simulink model "Adaptive_Cruise_Control"  (R2022b)
settings: configuration reference "CommonModelConfiguration" (kept outside this file)
undefined symbols (not defined in the file): cc_param_23, LCFG_ACC_IntStsDelay, LCFG_ACC_Tmr1, LCFG_ACC_Tmr2, LCFG_ActivationDeactivation, LCFG_DSF_Timeout
settings Model: Creator=rkallum  LastModifiedBy=OTHOMSO1
settings ConfigSetRef: SourceName=CommonModelConfiguration  SourceLocation=Base Workspace

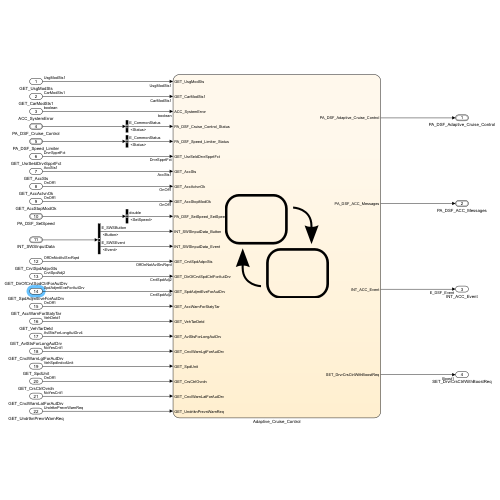
[thumbnail: Simulink's stored preview of the top-level diagram]
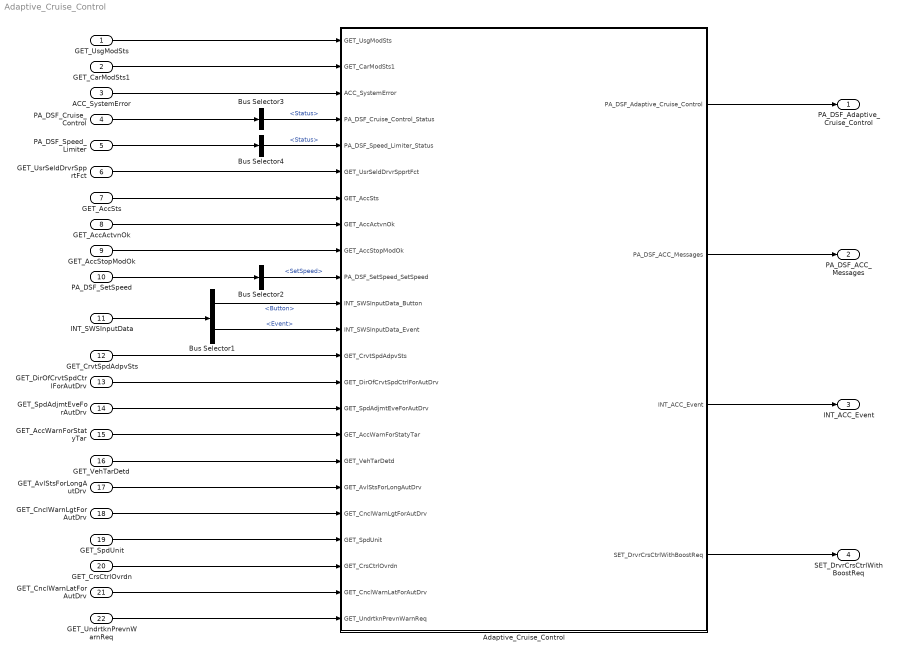
== system Adaptive_Cruise_Control ==
  GET_UsgModSts : Inport  OutDataTypeStr=Enum: UsgModSts1
  GET_CarModSts1 : Inport  Port=2  OutDataTypeStr=Enum: CarModSts1
  ACC_SystemError : Inport  Port=3  OutDataTypeStr=boolean
  PA_DSF_Cruise_Control : Inport  Port=4  OutDataTypeStr=Bus: PA_DSF
  PA_DSF_Speed_Limiter : Inport  Port=5  OutDataTypeStr=Bus: PA_DSF
  GET_UsrSeldDrvrSpprtFct : Inport  Port=6  OutDataTypeStr=Enum: DrvrSpprtFct
  GET_AccSts : Inport  Port=7  OutDataTypeStr=Enum: AccSts1
  GET_AccActvnOk : Inport  Port=8  OutDataTypeStr=Enum: OnOff1
  GET_AccStopModOk : Inport  Port=9  OutDataTypeStr=Enum: OnOff1
  PA_DSF_SetSpeed : Inport  Port=10  OutDataTypeStr=Bus: PA_StatusAndValueAndDoubleAndDouble
  INT_SWSInputData : Inport  Port=11  OutDataTypeStr=Bus: SWSInputData  LockScale=on
  GET_CrvtSpdAdpvSts : Inport  Port=12  OutDataTypeStr=Enum: OffOnNotAvlSrvRqrd
  GET_DirOfCrvtSpdCtrlForAutDrv : Inport  Port=13  OutDataTypeStr=Enum: CrvtSpdAdj2
  GET_SpdAdjmtEveForAutDrv : Inport  Port=14  OutDataTypeStr=Enum: SpdAdjmtEveForAutDrv
  GET_AccWarnForStatyTar : Inport  Port=15  OutDataTypeStr=Enum: OnOff1
  GET_VehTarDetd : Inport  Port=16  OutDataTypeStr=Enum: VehDetd1
  GET_AvlStsForLongAutDrv : Inport  Port=17  OutDataTypeStr=Enum: AvlStsForLongAutDrv4
  GET_CnclWarnLgtForAutDrv : Inport  Port=18  OutDataTypeStr=Enum: NoYesCrit1
  GET_SpdUnit : Inport  Port=19  OutDataTypeStr=Enum: VehSpdIndcdUnit
  GET_CrsCtrlOvrdn : Inport  Port=20  OutDataTypeStr=Enum: OnOff1
  GET_CnclWarnLatForAutDrv : Inport  Port=21  OutDataTypeStr=Enum: NoYesCrit1
  GET_UndrtknPrevnWarnReq : Inport  Port=22  OutDataTypeStr=Enum: UndrtknPrevnWarnReq
  Adaptive_Cruise_Control : Stateflow chart  TreatAsAtomicUnit=on
  Bus Selector1 : BusSelector  OutputSignals=Button,Event
  Bus Selector2 : BusSelector  OutputSignals=SetSpeed
  Bus Selector3 : BusSelector  OutputSignals=Status
  Bus Selector4 : BusSelector  OutputSignals=Status
  PA_DSF_Adaptive_Cruise_Control : Outport  OutDataTypeStr=Bus: PA_DSF_ACC  VectorParamsAs1DForOutWhenUnconnected=off
  PA_DSF_ACC_Messages : Outport  Port=2  OutDataTypeStr=Bus: PA_DSF_Message  VectorParamsAs1DForOutWhenUnconnected=off
  INT_ACC_Event : Outport  Port=3  OutDataTypeStr=Enum: E_DSF_Event  VectorParamsAs1DForOutWhenUnconnected=off
  SET_DrvrCrsCtrlWithBoostReq : Outport  Port=4  OutDataTypeStr=Enum: Boost1  VectorParamsAs1DForOutWhenUnconnected=off
  wires:
  ACC_SystemError/1 -> Adaptive_Cruise_Control/3(ACC_SystemError)
  PA_DSF_Cruise_Control/1 -> Bus Selector3/1
  PA_DSF_Speed_Limiter/1 -> Bus Selector4/1
  GET_UsrSeldDrvrSpprtFct/1 -> Adaptive_Cruise_Control/6(GET_UsrSeldDrvrSpprtFct)
  GET_AccSts/1 -> Adaptive_Cruise_Control/7(GET_AccSts)
  GET_AccActvnOk/1 -> Adaptive_Cruise_Control/8(GET_AccActvnOk)
  GET_AccStopModOk/1 -> Adaptive_Cruise_Control/9(GET_AccStopModOk)
  PA_DSF_SetSpeed/1 -> Bus Selector2/1
  GET_CrvtSpdAdpvSts/1 -> Adaptive_Cruise_Control/13(GET_CrvtSpdAdpvSts)
  GET_DirOfCrvtSpdCtrlForAutDrv/1 -> Adaptive_Cruise_Control/14(GET_DirOfCrvtSpdCtrlForAutDrv)
  GET_AccWarnForStatyTar/1 -> Adaptive_Cruise_Control/16(GET_AccWarnForStatyTar)
  GET_VehTarDetd/1 -> Adaptive_Cruise_Control/17(GET_VehTarDetd)
  GET_AvlStsForLongAutDrv/1 -> Adaptive_Cruise_Control/18(GET_AvlStsForLongAutDrv)
  GET_CnclWarnLgtForAutDrv/1 -> Adaptive_Cruise_Control/19(GET_CnclWarnLgtForAutDrv)
  GET_SpdUnit/1 -> Adaptive_Cruise_Control/20(GET_SpdUnit)
  Adaptive_Cruise_Control/3(INT_ACC_Event) -> INT_ACC_Event/1
  Adaptive_Cruise_Control/2(PA_DSF_ACC_Messages) -> PA_DSF_ACC_Messages/1
  Adaptive_Cruise_Control/1(PA_DSF_Adaptive_Cruise_Control) -> PA_DSF_Adaptive_Cruise_Control/1
  INT_SWSInputData/1 -> Bus Selector1/1
  Bus Selector1/2 -> Adaptive_Cruise_Control/12(INT_SWSInputData_Event)  "<Event>"
  Bus Selector1/1 -> Adaptive_Cruise_Control/11(INT_SWSInputData_Button)  "<Button>"
  Bus Selector2/1 -> Adaptive_Cruise_Control/10(PA_DSF_SetSpeed_SetSpeed)  "<SetSpeed>"
  Bus Selector3/1 -> Adaptive_Cruise_Control/4(PA_DSF_Cruise_Control_Status)  "<Status>"
  Bus Selector4/1 -> Adaptive_Cruise_Control/5(PA_DSF_Speed_Limiter_Status)  "<Status>"
  Adaptive_Cruise_Control/4(SET_DrvrCrsCtrlWithBoostReq) -> SET_DrvrCrsCtrlWithBoostReq/1
  GET_CrsCtrlOvrdn/1 -> Adaptive_Cruise_Control/21(GET_CrsCtrlOvrdn)
  GET_CnclWarnLatForAutDrv/1 -> Adaptive_Cruise_Control/22(GET_CnclWarnLatForAutDrv)
  GET_UndrtknPrevnWarnReq/1 -> Adaptive_Cruise_Control/23(GET_UndrtknPrevnWarnReq)
  GET_SpdAdjmtEveForAutDrv/1 -> Adaptive_Cruise_Control/15(GET_SpdAdjmtEveForAutDrv)
  GET_UsgModSts/1 -> Adaptive_Cruise_Control/1(GET_UsgModSts)
  GET_CarModSts1/1 -> Adaptive_Cruise_Control/2(GET_CarModSts1)

== stateflow chart Adaptive_Cruise_Control/Adaptive_Cruise_Control ==
  state CARCONFIG_INVALID
    entry:
    PA_DSF_Adaptive_Cruise_Control.Status=E_CommonStatus.NotPresent;
    PA_DSF_Adaptive_Cruise_Control.Value=E_DSF_Value.DSF_Selected;
    PA_DSF_Adaptive_Cruise_Control.Data=E_DSF_Data.DSF_NoTarget;
    PA_DSF_ACC_Messages.Status=E_CommonStatus.NotPresent;
    PA_DSF_ACC_Messages.Value=E_DSF_Messages.Messages_Off;
    SET_DrvrCrsCtrlWithBoostReq=Boost1.Boost1_NoBoost;
    INT_ACC_Event=E_DSF_Event.NoReq;
  state SYSTEM_OK
    state isActive = ActivationCheck [function]
      (default) -> (junction 24)
      (junction 24) -> (junction 32) [order 1] : [GET_CarModSts1==CarModSts1.CarModSts1_CarModNorm &&...
          | GET_UsgModSts==UsgModSts1.UsgModSts1_UsgModDrvg &&...
          | (GET_UsrSeldDrvrSpprtFct==DrvrSpprtFct.DrvrSpprtFct_ACC ||...
          | PA_DSF_Adaptive_Cruise_Control.Value==E_DSF_Value.DSF_Active) &&...
          | PA_DSF_Cruise_Control_Status~=E_CommonStatus.Available &&...
          | PA_DSF_Speed_Limiter_Status~=E_CommonStatus.Available]
      (junction 24) -> (junction 26) [order 2] : {isActive=false;}
      (junction 32) -> (junction 23) : {isActive=true;}
      (junction 23) -> (junction 26)
      (junction 26) -> (junction 28)
    state NOT_ACTIVE
      entry:
      PA_DSF_Adaptive_Cruise_Control.Status = E_CommonStatus.Disabled;
      PA_DSF_Adaptive_Cruise_Control.Data = E_DSF_Data.DSF_NoTarget;
      INT_ACC_Event = E_DSF_Event.NoReq;
      PA_DSF_ACC_Messages.Status = E_CommonStatus.Disabled;
      SET_DrvrCrsCtrlWithBoostReq = Boost1.Boost1_NoBoost;
      state NO_MESSAGES
        entry:
        PA_DSF_ACC_Messages.Value = E_DSF_Messages.Messages_Off;
        PA_DSF_Adaptive_Cruise_Control.Value = E_DSF_Value.DSF_Selected;
      state CANCEL_WARNING
        entry:
        PA_DSF_ACC_Messages.Value = E_DSF_Messages.Messages_CancelWarning;
        PA_DSF_Adaptive_Cruise_Control.Value = E_DSF_Value.DSF_Selected;
      (default) -> (junction 303)
      (junction 303) -> (junction 308) [order 1] : [PA_DSF_Adaptive_Cruise_Control.Value==E_DSF_Value.DSF_Active ||...
          | PA_DSF_Adaptive_Cruise_Control.Value==E_DSF_Value.DSF_StopMode]
      (junction 303) -> SYSTEM_OK.NOT_ACTIVE.NO_MESSAGES [order 2]
      (junction 308) -> SYSTEM_OK.NOT_ACTIVE.CANCEL_WARNING
      SYSTEM_OK.NOT_ACTIVE.CANCEL_WARNING -> SYSTEM_OK.NOT_ACTIVE.NO_MESSAGES : [after(LCFG_DSF_Timeout, sec)]
    state PENDING
    state PENDING1
    state ACTIVE
      state MESSAGES [parallel]
        entry:
        PA_DSF_ACC_Messages.Status = E_CommonStatus.Available;
        settings: executionOrder=1
        state retVal = accMessages [function]
          state retVal2 = accActivationReq [function]
            (default) -> (junction 631)
            (junction 631) -> (junction 632) [order 1] : [(INT_SWSInputData_Button==E_SWSButton.BtnL5Req &&...
                | hasChangedTo(INT_SWSInputData_Event, E_SWSEvent.Push) &&...
                | PA_DSF_SetSpeed_SetSpeed~=0) &&...
                | GET_AccActvnOk==OnOff1.OnOff1_Off &&...
                | (GET_AccSts == AccSts1.AccSts1_Off ||...
                | GET_AccSts == AccSts1.AccSts1_Stb)]
            (junction 631) -> (junction 633) [order 2]
            (junction 632) -> (junction 634)
            (junction 633) -> (junction 634) [order 1] : [INT_SWSInputData_Button==E_SWSButton.BtnL1Req &&...
                | hasChangedTo(INT_SWSInputData_Event, E_SWSEvent.Push) &&...
                | GET_AccActvnOk==OnOff1.OnOff1_Off &&...
                | (GET_AccSts == AccSts1.AccSts1_Off ||...
                | GET_AccSts == AccSts1.AccSts1_Stb)]
            (junction 633) -> (junction 635) [order 2]
            (junction 634) -> (junction 636)
            (junction 635) -> (junction 636) [order 1] : [INT_SWSInputData_Button==E_SWSButton.BtnL5Req &&...
                | hasChangedTo(INT_SWSInputData_Event, E_SWSEvent.Push) &&...
                | PA_DSF_Adaptive_Cruise_Control.Value==E_DSF_Value.DSF_StopMode]
            (junction 635) -> (junction 637) [order 2] : {retVal2=false;}
            (junction 636) -> (junction 638) : {retVal2=true;}
            (junction 638) -> (junction 637)
            (junction 637) -> (junction 639)
          (default) -> (junction 432)
          (junction 432) -> (junction 433) [order 1] : [accActivationReq()]
          (junction 433) -> (junction 436) [order 1] : [(GET_AvlStsForLongAutDrv== AvlStsForLongAutDrv4.AvlStsForLongAutDrv4_LgtCtrlNotAvl ||...
              | GET_AvlStsForLongAutDrv==AvlStsForLongAutDrv4.AvlStsForLongAutDrv4_AccCncl)]
              | {PA_DSF_ACC_Messages.Value = E_DSF_Messages.Messages_Unavailable;}
          (junction 432) -> (junction 483) [order 2]
          (junction 433) -> (junction 438) [order 2]
          (junction 436) -> (junction 440)
          (junction 438) -> (junction 440) [order 1] : [(GET_AvlStsForLongAutDrv==AvlStsForLongAutDrv4.AvlStsForLongAutDrv4_NoVehAhd) &&...
              | (GET_SpdUnit==VehSpdIndcdUnit.VehSpdIndcdUnit_Kmph)]
              | {PA_DSF_ACC_Messages.Value = E_DSF_Messages.Messages_UnavailableBelow30kph;}
          (junction 438) -> (junction 443) [order 2]
          (junction 440) -> (junction 445)
          (junction 443) -> (junction 445) [order 1] : [(GET_AvlStsForLongAutDrv==AvlStsForLongAutDrv4.AvlStsForLongAutDrv4_DrvrBucdRqrd)]
              | {PA_DSF_ACC_Messages.Value = E_DSF_Messages.Messages_UnavailableUnbuckled;}
          (junction 443) -> (junction 448) [order 2]
          (junction 445) -> (junction 450)
          (junction 448) -> (junction 450) [order 1] : [(GET_AvlStsForLongAutDrv==AvlStsForLongAutDrv4.AvlStsForLongAutDrv4_DrvrDoorNotClsd)]
              | {PA_DSF_ACC_Messages.Value = E_DSF_Messages.Messages_UnavailableDoorOpen;}
          (junction 448) -> (junction 453) [order 2]
          (junction 450) -> (junction 455)
          (junction 453) -> (junction 455) [order 1] : [(GET_AvlStsForLongAutDrv==AvlStsForLongAutDrv4.AvlStsForLongAutDrv4_EpbAppld)]
              | {PA_DSF_ACC_Messages.Value = E_DSF_Messages.Messages_UnavailableEPB;}
          (junction 453) -> (junction 458) [order 2]
          (junction 455) -> (junction 460)
          (junction 458) -> (junction 460) [order 1] : [(GET_AvlStsForLongAutDrv==AvlStsForLongAutDrv4.AvlStsForLongAutDrv4_NoVehAhd) &&...
              | (GET_SpdUnit==VehSpdIndcdUnit.VehSpdIndcdUnit_Mph)]
              | {PA_DSF_ACC_Messages.Value = E_DSF_Messages.Messages_UnavailableBelow20mph;}
          (junction 458) -> (junction 463) [order 2]
          (junction 460) -> (junction 465)
          (junction 463) -> (junction 465) [order 1] : [(GET_AvlStsForLongAutDrv==AvlStsForLongAutDrv4.AvlStsForLongAutDrv4_GearNotInDrv)]
              | {PA_DSF_ACC_Messages.Value = E_DSF_Messages.Messages_UnavailableGear;}
          (junction 463) -> (junction 468) [order 2]
          (junction 465) -> (junction 470)
          (junction 468) -> (junction 470) [order 1] : [(GET_AvlStsForLongAutDrv==AvlStsForLongAutDrv4.AvlStsForLongAutDrv4_SnsrBlkd)]
              | {PA_DSF_ACC_Messages.Value = E_DSF_Messages.Messages_UnavailableSensor;}
          (junction 468) -> (junction 473) [order 2]
          (junction 470) -> (junction 475)
          (junction 473) -> (junction 475) [order 1] : [(GET_AvlStsForLongAutDrv==AvlStsForLongAutDrv4.AvlStsForLongAutDrv4_SpdLowLimExcdd)]
              | {PA_DSF_ACC_Messages.Value = E_DSF_Messages.Messages_UnavailableLowSpeed;}
          (junction 473) -> (junction 478) [order 2]
          (junction 475) -> (junction 480)
          (junction 478) -> (junction 483) [order 2]
          (junction 478) -> (junction 480) [order 1] : [(GET_AvlStsForLongAutDrv==AvlStsForLongAutDrv4.AvlStsForLongAutDrv4_DrvModSeldNotOk)]
              | {PA_DSF_ACC_Messages.Value = E_DSF_Messages.Messages_UnavailableDriveMode;}
          (junction 483) -> (junction 486)
          (junction 480) -> (junction 490)
          (junction 486) -> (junction 488) [order 1] : [GET_CnclWarnLgtForAutDrv==NoYesCrit1.NoYesCrit1_Yes ||...
              | GET_CnclWarnLatForAutDrv==NoYesCrit1.NoYesCrit1_Yes]
          (junction 488) -> (junction 490) [order 1] : [hasChangedTo(GET_AvlStsForLongAutDrv, AvlStsForLongAutDrv4.AvlStsForLongAutDrv4_SnsrBlkd)]
              | {PA_DSF_ACC_Messages.Value = E_DSF_Messages.Messages_CancelSensor;}
          (junction 486) -> (junction 522) [order 2]
          (junction 488) -> (junction 492) [order 2]
          (junction 490) -> (junction 494)
          (junction 492) -> (junction 494) [order 1] : [hasChangedTo(GET_AvlStsForLongAutDrv, AvlStsForLongAutDrv4.AvlStsForLongAutDrv4_HldTiMaxExcdd)]
              | {PA_DSF_ACC_Messages.Value = E_DSF_Messages.Messages_CancelMaxHold;}
          (junction 492) -> (junction 497) [order 2]
          (junction 494) -> (junction 499)
          (junction 497) -> (junction 499) [order 1] : [hasChangedTo(GET_AvlStsForLongAutDrv, AvlStsForLongAutDrv4.AvlStsForLongAutDrv4_SpdLowLimExcdd)]
              | {PA_DSF_ACC_Messages.Value = E_DSF_Messages.Messages_CancelLowSpeed;}
          (junction 497) -> (junction 502) [order 2]
          (junction 499) -> (junction 504)
          (junction 502) -> (junction 504) [order 1] : [hasChangedTo(GET_AvlStsForLongAutDrv, AvlStsForLongAutDrv4.AvlStsForLongAutDrv4_DrvModSeldNotOk)]
              | {PA_DSF_ACC_Messages.Value = E_DSF_Messages.Messages_CancelDriveMode;}
          (junction 502) -> (junction 507) [order 2]
          (junction 504) -> (junction 509)
          (junction 507) -> (junction 509) [order 1] : [hasChangedTo(GET_AvlStsForLongAutDrv, AvlStsForLongAutDrv4.AvlStsForLongAutDrv4_LgtCtrlNotAvl) || ...
              | hasChangedTo(GET_AvlStsForLongAutDrv, AvlStsForLongAutDrv4.AvlStsForLongAutDrv4_AccCncl)]
              | {PA_DSF_ACC_Messages.Value = E_DSF_Messages.Messages_CancelWarning;}
          (junction 507) -> (junction 511) [order 2]
          (junction 509) -> (junction 513)
          (junction 511) -> (junction 513) [order 1] : [hasChangedTo(GET_AvlStsForLongAutDrv, AvlStsForLongAutDrv4.AvlStsForLongAutDrv4_NoVehAhd)]
              | {PA_DSF_ACC_Messages.Value = E_DSF_Messages.Messages_CancelNoLeadVehicle;}
          (junction 511) -> (junction 515) [order 2]
          (junction 513) -> (junction 517)
          (junction 515) -> (junction 522) [order 2]
          (junction 515) -> (junction 517) [order 1] : [hasChangedTo(GET_AvlStsForLongAutDrv, AvlStsForLongAutDrv4.AvlStsForLongAutDrv4_OvrdTiMaxExcdd)]
              | {PA_DSF_ACC_Messages.Value = E_DSF_Messages.Messages_CancelMaxOverride;}
          (junction 522) -> (junction 525) : {retVal = false;}
          (junction 517) -> (junction 527) : {retVal = true;}
          (junction 527) -> (junction 525)
          (junction 525) -> (junction 530)
        state HIDE_MESSAGES
          entry: PA_DSF_ACC_Messages.Value = E_DSF_Messages.Messages_Off;
        state SHOW_MESSAGES
        (default) -> HIDE_MESSAGES
        HIDE_MESSAGES -> SHOW_MESSAGES : [accMessages()]
        SHOW_MESSAGES -> HIDE_MESSAGES [order 2] : [hasChangedTo(GET_AccSts, AccSts1.AccSts1_Actv) ||...
            | hasChangedTo(GET_AccSts, AccSts1.AccSts1_Stop) ||...
            | after(LCFG_DSF_Timeout, sec)]
        SHOW_MESSAGES -> SHOW_MESSAGES [order 1] : [accMessages()]
      state ACC [parallel]
        entry: PA_DSF_Adaptive_Cruise_Control.Status = E_CommonStatus.Available;
        settings: executionOrder=2
        state STANDBY
          entry:
          PA_DSF_Adaptive_Cruise_Control.Value = E_DSF_Value.DSF_Standby;
          PA_DSF_Adaptive_Cruise_Control.Data = E_DSF_Data.DSF_NoTarget;
          state NEW_EVENT_POSSIBLE
            entry: INT_ACC_Event=E_DSF_Event.NoReq;
          state EVENT_IN_PROGRESS
          (default) -> SYSTEM_OK.ACTIVE.ACC.STANDBY.EVENT_IN_PROGRESS
          SYSTEM_OK.ACTIVE.ACC.STANDBY.EVENT_IN_PROGRESS -> SYSTEM_OK.ACTIVE.ACC.STANDBY.NEW_EVENT_POSSIBLE : [after(LCFG_ActivationDeactivation,sec)]
        state SELECTED
          entry: PA_DSF_Adaptive_Cruise_Control.Value = E_DSF_Value.DSF_Selected;
        state ON
          state ACC_ACTIVE
            entry: PA_DSF_Adaptive_Cruise_Control.Value = E_DSF_Value.DSF_Active;
            entry, during: activeData();
            state NEW_EVENT_POSSIBLE
              entry: INT_ACC_Event = E_DSF_Event.NoReq;
            state EVENT_IN_PROGRESS
            state activeData [function]
              (default) -> (junction 674)
              (junction 674) -> (junction 678) [order 1] : [GET_CrsCtrlOvrdn==OnOff1.OnOff1_On]
                  | {PA_DSF_Adaptive_Cruise_Control.Data = E_DSF_Data.DSF_CruiseOverridden;}
              (junction 674) -> (junction 151) [order 2]
              (junction 678) -> (junction 153)
              (junction 151) -> (junction 153) [order 1] : [GET_CrvtSpdAdpvSts== OffOnNotAvlSrvRqrd.OffOnNotAvlSrvRqrd_On &&...
                  | GET_DirOfCrvtSpdCtrlForAutDrv==CrvtSpdAdj2.CrvtSpdAdj2_CrvtSpdAdpvLe]
                  | {PA_DSF_Adaptive_Cruise_Control.Data = E_DSF_Data.DSF_CSA_Left;}
              (junction 151) -> (junction 161) [order 2]
              (junction 153) -> (junction 154)
              (junction 161) -> (junction 154) [order 1] : [GET_CrvtSpdAdpvSts==OffOnNotAvlSrvRqrd.OffOnNotAvlSrvRqrd_On &&...
                  | GET_DirOfCrvtSpdCtrlForAutDrv==CrvtSpdAdj2.CrvtSpdAdj2_CrvtSpdAdpvRi]
                  | {PA_DSF_Adaptive_Cruise_Control.Data = E_DSF_Data.DSF_CSA_Right;}
              (junction 161) -> (junction 719) [order 2]
              (junction 154) -> (junction 723)
              (junction 719) -> (junction 723) [order 1] : [GET_CrvtSpdAdpvSts==OffOnNotAvlSrvRqrd.OffOnNotAvlSrvRqrd_On &&...
                  | GET_SpdAdjmtEveForAutDrv==SpdAdjmtEveForAutDrv.SpdAdjmtEveForAutDrv_HighwayExitLeft]
                  | {PA_DSF_Adaptive_Cruise_Control.Data = E_DSF_Data.DSF_CSA_ExitLeft;}
              (junction 719) -> (junction 720) [order 2]
              (junction 723) -> (junction 727)
              (junction 720) -> (junction 727) [order 1] : [GET_CrvtSpdAdpvSts==OffOnNotAvlSrvRqrd.OffOnNotAvlSrvRqrd_On &&...
                  | GET_SpdAdjmtEveForAutDrv==SpdAdjmtEveForAutDrv.SpdAdjmtEveForAutDrv_HighwayExitRight]
                  | {PA_DSF_Adaptive_Cruise_Control.Data = E_DSF_Data.DSF_CSA_ExitRight;}
              (junction 720) -> (junction 721) [order 2]
              (junction 727) -> (junction 730)
              (junction 721) -> (junction 730) [order 1] : [GET_CrvtSpdAdpvSts==OffOnNotAvlSrvRqrd.OffOnNotAvlSrvRqrd_On &&...
                  | (GET_SpdAdjmtEveForAutDrv==SpdAdjmtEveForAutDrv.SpdAdjmtEveForAutDrv_Roundabout ||...
                  | GET_DirOfCrvtSpdCtrlForAutDrv==CrvtSpdAdj2.CrvtSpdAdj2_CrvtSpdAdpvOtherObj)]
                  | {PA_DSF_Adaptive_Cruise_Control.Data = E_DSF_Data.DSF_CSA_Roundabout;}
              (junction 721) -> (junction 735) [order 2]
              (junction 730) -> (junction 737)
              (junction 735) -> (junction 737) [order 1] : [GET_CrvtSpdAdpvSts==OffOnNotAvlSrvRqrd.OffOnNotAvlSrvRqrd_On &&...
                  | GET_SpdAdjmtEveForAutDrv==SpdAdjmtEveForAutDrv.SpdAdjmtEveForAutDrv_Intersection]
                  | {PA_DSF_Adaptive_Cruise_Control.Data = E_DSF_Data.DSF_CSA_Intersection;}
              (junction 735) -> (junction 157) [order 2]
              (junction 737) -> (junction 156)
              (junction 157) -> (junction 156) [order 1] : [GET_AccWarnForStatyTar==OnOff1.OnOff1_On]
                  | {PA_DSF_Adaptive_Cruise_Control.Data = E_DSF_Data.DSF_StationaryTarget;}
              (junction 157) -> (junction 708) [order 2]
              (junction 156) -> (junction 709)
              (junction 708) -> (junction 709) [order 1] : [GET_UndrtknPrevnWarnReq==UndrtknPrevnWarnReq.UndrtknPrevnWarnReq_WarnForUndrtknPrevnLe]
                  | {PA_DSF_Adaptive_Cruise_Control.Data = E_DSF_Data.DSF_UndertakePrevention_Left;}
              (junction 708) -> (junction 710) [order 2]
              (junction 709) -> (junction 711)
              (junction 710) -> (junction 711) [order 1] : [GET_UndrtknPrevnWarnReq==UndrtknPrevnWarnReq.UndrtknPrevnWarnReq_WarnForUndrtknPrevnRi]
                  | {PA_DSF_Adaptive_Cruise_Control.Data = E_DSF_Data.DSF_UndertakePrevention_Right;}
              (junction 710) -> (junction 160) [order 2]
              (junction 711) -> (junction 159)
              (junction 160) -> (junction 159) [order 1] : [GET_VehTarDetd~= VehDetd1.VehDetd1_NoVehDetd]
                  | {PA_DSF_Adaptive_Cruise_Control.Data = E_DSF_Data.DSF_Target;}
              (junction 160) -> (junction 158) [order 2] : {PA_DSF_Adaptive_Cruise_Control.Data = E_DSF_Data.DSF_NoTarget;}
              (junction 159) -> (junction 187)
              (junction 187) -> (junction 158)
              (junction 158) -> (junction 188)
            (default) -> SYSTEM_OK.ACTIVE.ACC.ON.ACC_ACTIVE.EVENT_IN_PROGRESS
            SYSTEM_OK.ACTIVE.ACC.ON.ACC_ACTIVE.EVENT_IN_PROGRESS -> SYSTEM_OK.ACTIVE.ACC.ON.ACC_ACTIVE.NEW_EVENT_POSSIBLE : [after(LCFG_ActivationDeactivation,sec)]
            SYSTEM_OK.ACTIVE.ACC.ON.ACC_ACTIVE.NEW_EVENT_POSSIBLE -> SYSTEM_OK.ACTIVE.ACC.ON.ACC_ACTIVE.EVENT_IN_PROGRESS : [INT_SWSInputData_Button==E_SWSButton.BtnL5Req &&...
                | hasChangedTo(INT_SWSInputData_Event, E_SWSEvent.Push) &&...
                | GET_AccSts==AccSts1.AccSts1_StopTmp]
                | {INT_ACC_Event = E_DSF_Event.Resume;}
          state ACC_STOP
            entry: PA_DSF_Adaptive_Cruise_Control.Value = E_DSF_Value.DSF_StopMode;
            entry, during: stopData();
            state EVENT_IN_PROGRESS
            state NEW_EVENT_POSSIBLE
              entry: INT_ACC_Event = E_DSF_Event.NoReq;
            state stopData [function]
              (default) -> (junction 681)
              (junction 681) -> (junction 683) [order 1] : [GET_CrsCtrlOvrdn==OnOff1.OnOff1_On]
                  | {PA_DSF_Adaptive_Cruise_Control.Data = E_DSF_Data.DSF_NoTarget;}
              (junction 681) -> (junction 668) [order 2]
              (junction 683) -> (junction 670)
              (junction 668) -> (junction 670) [order 1] : [GET_AccWarnForStatyTar==OnOff1.OnOff1_On]
                  | {PA_DSF_Adaptive_Cruise_Control.Data = E_DSF_Data.DSF_StationaryTarget;}
              (junction 668) -> (junction 202) [order 2]
              (junction 670) -> (junction 203)
              (junction 202) -> (junction 203) [order 1] : [GET_VehTarDetd~=VehDetd1.VehDetd1_NoVehDetd]
                  | {PA_DSF_Adaptive_Cruise_Control.Data = E_DSF_Data.DSF_Target;}
              (junction 202) -> (junction 204) [order 2] : {PA_DSF_Adaptive_Cruise_Control.Data = E_DSF_Data.DSF_NoTarget;}
              (junction 203) -> (junction 205)
              (junction 205) -> (junction 204)
              (junction 204) -> (junction 206)
            (default) -> SYSTEM_OK.ACTIVE.ACC.ON.ACC_STOP.EVENT_IN_PROGRESS
            SYSTEM_OK.ACTIVE.ACC.ON.ACC_STOP.EVENT_IN_PROGRESS -> SYSTEM_OK.ACTIVE.ACC.ON.ACC_STOP.NEW_EVENT_POSSIBLE : [after(LCFG_ActivationDeactivation,sec)]
          (default) -> (junction 71)
          (junction 71) -> ACC_ACTIVE [order 1] : [GET_AccActvnOk==OnOff1.OnOff1_On]
          (junction 71) -> ACC_STOP [order 2]
          ACC_ACTIVE -> ACC_STOP : [(after(LCFG_ACC_IntStsDelay, sec) && GET_AccSts==AccSts1.AccSts1_Stop)]
          ACC_STOP -> ACC_ACTIVE [order 1] : [INT_SWSInputData_Button==E_SWSButton.BtnL5Req &&...
              | hasChangedTo(INT_SWSInputData_Event, E_SWSEvent.Push) &&...
              | GET_AccActvnOk==OnOff1.OnOff1_On]
              | {INT_ACC_Event=E_DSF_Event.Resume;}
          ACC_STOP -> ACC_ACTIVE [order 2] : [after(LCFG_ACC_IntStsDelay, sec) && GET_AccSts~=AccSts1.AccSts1_Stop]
        (default) -> SELECTED
        SELECTED -> ON [order 1] : [(INT_SWSInputData_Button==E_SWSButton.BtnL1Req &&...
            | hasChangedTo(INT_SWSInputData_Event, E_SWSEvent.Push) &&...
            | (GET_AccActvnOk==OnOff1.OnOff1_On ||...
            | GET_AccStopModOk==OnOff1.OnOff1_On))]
            | {INT_ACC_Event=E_DSF_Event.Activation;}
        SELECTED -> ON [order 2] : [after(LCFG_ACC_IntStsDelay, sec) &&...
            | GET_AccSts~=AccSts1.AccSts1_Off &&...
            | GET_AccSts~=AccSts1.AccSts1_Stb]
        STANDBY -> ON [order 1] : [(INT_SWSInputData_Button==E_SWSButton.BtnL5Req &&...
            | hasChangedTo(INT_SWSInputData_Event, E_SWSEvent.Push) &&...
            | (PA_DSF_SetSpeed_SetSpeed~=0) &&...
            | (GET_AccActvnOk==OnOff1.OnOff1_On ||...
            | GET_AccStopModOk==OnOff1.OnOff1_On) &&...
            | INT_ACC_Event==E_DSF_Event.NoReq)]
            | {INT_ACC_Event = E_DSF_Event.Resume;}
        STANDBY -> ON [order 2] : [(INT_SWSInputData_Button==E_SWSButton.BtnL1Req &&...
            | hasChangedTo(INT_SWSInputData_Event, E_SWSEvent.Push) &&...
            | (GET_AccActvnOk==OnOff1.OnOff1_On ||...
            | GET_AccStopModOk==OnOff1.OnOff1_On) &&...
            | INT_ACC_Event==E_DSF_Event.NoReq)]
            | {INT_ACC_Event = E_DSF_Event.Activation;}
        STANDBY -> ON [order 3] : [after(LCFG_ACC_IntStsDelay, sec) &&...
            | GET_AccSts~=AccSts1.AccSts1_Off &&...
            | GET_AccSts~=AccSts1.AccSts1_Stb]
        ON -> STANDBY [order 1] : [(INT_SWSInputData_Button==E_SWSButton.BtnL1Req &&...
            | hasChangedTo(INT_SWSInputData_Event, E_SWSEvent.Push)) ||...
            | INT_SWSInputData_Event==E_SWSEvent.Deactivation]
            | {INT_ACC_Event = E_DSF_Event.Deactivation;}
        ON -> STANDBY [order 2] : [(after(LCFG_ACC_IntStsDelay, sec) &&...
            | (GET_AccSts==AccSts1.AccSts1_Off ||...
            | GET_AccSts==AccSts1.AccSts1_Stb))]
      state ACC_BOOST [parallel]
        settings: executionOrder=3
        state NOREQ
          entry: SET_DrvrCrsCtrlWithBoostReq=Boost1.Boost1_NoBoost;
        state BOOST
          entry: SET_DrvrCrsCtrlWithBoostReq=Boost1.Boost1_BoostPos;
        (default) -> NOREQ
        BOOST -> NOREQ : [INT_SWSInputData_Button~=E_SWSButton.BtnL5Req ||...
            | INT_SWSInputData_Event==E_SWSEvent.Idle]
        NOREQ -> BOOST : [INT_SWSInputData_Button==E_SWSButton.BtnL5Req &&...
            | INT_SWSInputData_Event~=E_SWSEvent.Idle]
    (default) -> NOT_ACTIVE
    NOT_ACTIVE -> PENDING : [ActivationCheck()]
    PENDING -> NOT_ACTIVE [order 1] : [~ActivationCheck()]
    PENDING1 -> NOT_ACTIVE [order 1] : [after(LCFG_ACC_Tmr1,sec)]
    PENDING -> ACTIVE [order 2] : [after(LCFG_ACC_Tmr2,sec)]
    PENDING1 -> ACTIVE [order 2] : [ActivationCheck()]
    ACTIVE -> PENDING1 : [~ActivationCheck()]
  state SYSTEM_ERROR
    entry:
    PA_DSF_Adaptive_Cruise_Control.Status=E_CommonStatus.SystemError;
    PA_DSF_Adaptive_Cruise_Control.Data=E_DSF_Data.DSF_NoTarget;
    INT_ACC_Event=E_DSF_Event.NoReq;
    PA_DSF_ACC_Messages.Status=E_CommonStatus.SystemError;
    SET_DrvrCrsCtrlWithBoostReq=Boost1.Boost1_NoBoost;
    state retVal = accActivationReq [function]
      (default) -> (junction 615)
      (junction 615) -> (junction 616) [order 1] : [(INT_SWSInputData_Button==E_SWSButton.BtnL1Req ||...
          | INT_SWSInputData_Button==E_SWSButton.BtnL5Req) &&...
          | hasChangedTo(INT_SWSInputData_Event, E_SWSEvent.Push) &&...
          | GET_UsrSeldDrvrSpprtFct==DrvrSpprtFct.DrvrSpprtFct_ACC]
      (junction 615) -> (junction 620) [order 2] : {retVal=false;}
      (junction 616) -> (junction 618) : {retVal=true;}
      (junction 618) -> (junction 620)
      (junction 620) -> (junction 623)
    state CANCEL_WARNING
      entry:
      PA_DSF_ACC_Messages.Value=E_DSF_Messages.Messages_CancelWarning;
      PA_DSF_Adaptive_Cruise_Control.Value=E_DSF_Value.DSF_Selected;
    state UNAVAILABLE
      entry:
      PA_DSF_ACC_Messages.Value=E_DSF_Messages.Messages_Unavailable;
    state NO_MESSAGES
      entry:
      PA_DSF_ACC_Messages.Value=E_DSF_Messages.Messages_Off;
      PA_DSF_Adaptive_Cruise_Control.Value=E_DSF_Value.DSF_Selected;
    (default) -> (junction 558)
    (junction 558) -> (junction 557) [order 1] : [PA_DSF_Adaptive_Cruise_Control.Value==E_DSF_Value.DSF_Active ||...
        | PA_DSF_Adaptive_Cruise_Control.Value==E_DSF_Value.DSF_StopMode]
    (junction 558) -> SYSTEM_ERROR.NO_MESSAGES [order 2]
    (junction 557) -> SYSTEM_ERROR.CANCEL_WARNING
    UNAVAILABLE -> UNAVAILABLE [order 2] : [accActivationReq()]
    SYSTEM_ERROR.CANCEL_WARNING -> UNAVAILABLE [order 2] : [accActivationReq()]
    UNAVAILABLE -> SYSTEM_ERROR.NO_MESSAGES [order 1] : [after(LCFG_DSF_Timeout, sec)]
    SYSTEM_ERROR.NO_MESSAGES -> UNAVAILABLE : [accActivationReq()]
    SYSTEM_ERROR.CANCEL_WARNING -> SYSTEM_ERROR.NO_MESSAGES [order 1] : [after(LCFG_DSF_Timeout, sec)]
  (default) -> (junction 45)
  (junction 45) -> CARCONFIG_INVALID [order 2]
  (junction 45) -> (junction 49) [order 1] : [cc_param_23>2]
      | {PA_DSF_Adaptive_Cruise_Control.Value =...
      | E_DSF_Value.DSF_Selected;}
  (junction 49) -> SYSTEM_OK [order 2]
  (junction 49) -> (junction 51) [order 1] : [ACC_SystemError==1 ||...
      | INT_SWSInputData_Event==E_SWSEvent.ButtonStuck]
  SYSTEM_ERROR -> SYSTEM_OK : [ACC_SystemError==0 &&...
      | INT_SWSInputData_Event~=E_SWSEvent.ButtonStuck]
  SYSTEM_OK -> SYSTEM_ERROR : [ACC_SystemError==1 ||...
      | INT_SWSInputData_Event==E_SWSEvent.ButtonStuck]
      | {INT_ACC_Event=E_DSF_Event.Deactivation;}
  (junction 51) -> SYSTEM_ERROR
  data: isActive function_output boolean; retVal2 function_output; retVal function_output; retVal function_output; cc_param_23 parameter; GET_UsgModSts input Enum: UsgModSts1; GET_CarModSts1 input Enum: CarModSts1; ACC_SystemError input boolean; PA_DSF_Cruise_Control_Status input Enum: E_CommonStatus; PA_DSF_Speed_Limiter_Status input Enum: E_CommonStatus; LCFG_ACC_Tmr1 parameter; LCFG_ACC_Tmr2 parameter; GET_UsrSeldDrvrSpprtFct input Enum: DrvrSpprtFct; PA_DSF_Adaptive_Cruise_Control output Bus: PA_DSF_ACC =0; PA_DSF_ACC_Messages output Bus: PA_DSF_Message =0; GET_AccSts input Enum: AccSts1; GET_AccActvnOk input Enum: OnOff1; GET_AccStopModOk input Enum: OnOff1; INT_ACC_Event output Enum: E_DSF_Event; PA_DSF_SetSpeed_SetSpeed input double; LCFG_ACC_IntStsDelay parameter; INT_SWSInputData_Button input Enum: E_SWSButton; INT_SWSInputData_Event input Enum: E_SWSEvent; GET_CrvtSpdAdpvSts input Enum: OffOnNotAvlSrvRqrd; GET_DirOfCrvtSpdCtrlForAutDrv input Enum: CrvtSpdAdj2; GET_SpdAdjmtEveForAutDrv input; GET_AccWarnForStatyTar input Enum: OnOff1; GET_VehTarDetd input Enum: VehDetd1; GET_AvlStsForLongAutDrv input Enum: AvlStsForLongAutDrv4; GET_CnclWarnLgtForAutDrv input Enum: NoYesCrit1; GET_SpdUnit input Enum: VehSpdIndcdUnit; LCFG_DSF_Timeout parameter; SET_DrvrCrsCtrlWithBoostReq output Enum: Boost1; GET_CrsCtrlOvrdn input Enum: OnOff1; LCFG_ActivationDeactivation parameter; GET_CnclWarnLatForAutDrv input Enum: NoYesCrit1; GET_UndrtknPrevnWarnReq input Enum: UndrtknPrevnWarnReq
